simulink model "proj6_week1"  (R2021a)
settings: Solver=VariableStepAuto  StartTime=0.0  StopTime=10.0  RelTol=1e-3
settings Model: Creator=RASIKA MALGI  LastModifiedBy=RASIKA MALGI
settings SolverCC: AlgebraicLoopSolver=TrustRegion
settings DebuggingCC: SFMachineParentedDataDiag=warning

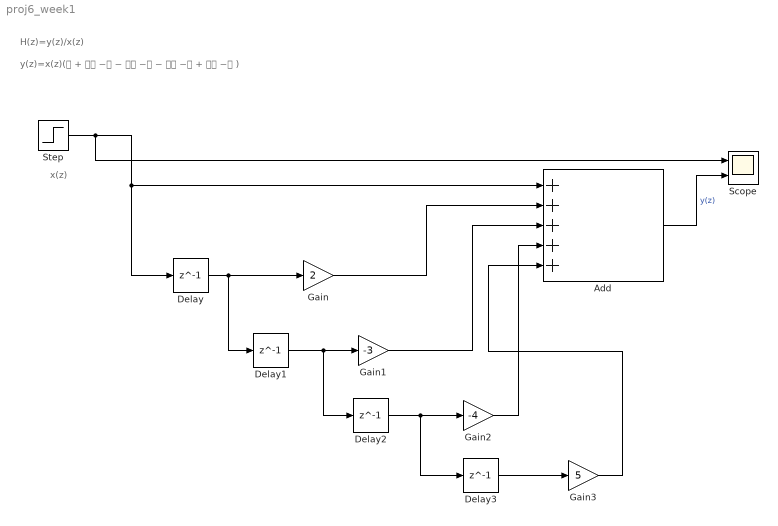
== system proj6_week1 ==
  note: y(z)=x(z)(𝟏 + 𝟐𝐳 −𝟏 − 𝟑𝐳 −𝟐 − 𝟒𝐳 −𝟑 + 𝟓𝐳 −𝟒 )
  note: H(z)=y(z)/x(z)
  note: x(z)
  Add : Sum  Inputs=+++++
  Delay{,1..3} (4 alike) : Delay  DelayLength=1  InitialCondition=0
  Gain : Gain  Gain=2
  Gain1 : Gain  Gain=-3
  Gain2 : Gain  Gain=-4
  Gain3 : Gain  Gain=5
  Scope : Scope  NumInputPorts=2
  Step : Step  SampleTime=0
  wires:
  Delay/1 -> Delay1/1, Gain/1
  Delay1/1 -> Delay2/1, Gain1/1
  Delay2/1 -> Delay3/1, Gain2/1
  Delay3/1 -> Gain3/1
  Step/1 -> Scope/1, Delay/1, Add/1
  Gain/1 -> Add/2
  Gain1/1 -> Add/3
  Gain2/1 -> Add/4
  Gain3/1 -> Add/5
  Add/1 -> Scope/2  "y(z)"
